simulink model "simulation"  (Simulink 8.1)
settings: Solver=ode45  StartTime=0.0  StopTime=max(t_simulink)  RelTol=1e-3
values from neighbouring files (symbols this model uses):
  fe_simulink = 50000    [TP.m]
libraries: librairie x6
settings Model: Creator=sylar  LastModifiedBy=tung  SimulationMode=accelerator
settings DebuggingCC: StrictBusMsg=Warning

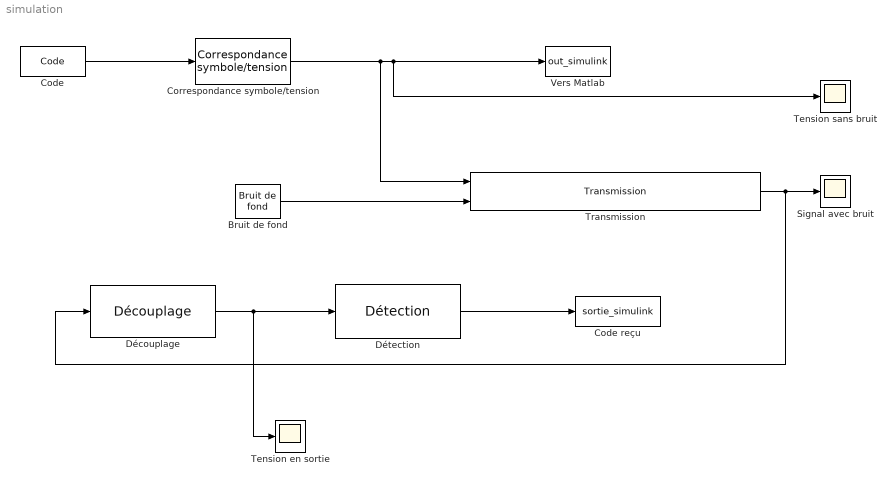
== system simulation ==
  Bruit de fond : librairie/Bruit de fond  RSB=-15
  Code : librairie/Code  T_symbole=Tsymbole_simulink
  Code reçu : ToWorkspace  VariableName=sortie_simulink  SampleTime=-1
  Correspondance symbole/tension : librairie/Correspondance symbole//tension  A_symbole=5
  Découplage : librairie/Découplage  TOTO=0
  Détection : librairie/Détection  seuil=0
  "Signal avec bruit " : Scope
      settings: YMin=-7  YMax=8
  Tension en sortie : Scope
      settings: YMin=-7  YMax=8  SaveName=ScopeData2
  "Tension sans bruit " : Scope
      settings: YMin=-7  YMax=8
  Transmission : librairie/Transmission  TOTO=[]
  Vers Matlab : ToWorkspace  VariableName=out_simulink  SampleTime=1/fe_simulink
  wires:
  Code/1 -> Correspondance symbole/tension/1
  Correspondance symbole/tension/1 -> Transmission/1, "Tension sans bruit "/1, Vers Matlab/1
  Transmission/1 -> Découplage/1, "Signal avec bruit "/1
  Bruit de fond/1 -> Transmission/2
  Découplage/1 -> Tension en sortie/1, Détection/1
  Détection/1 -> Code reçu/1
